simulink model "Ports"  (Simulink 7.4)
settings: Solver=ode45  StartTime=0.0  StopTime=10.0  RelTol=1e-3
settings Model: Creator=dread  LastModifiedBy=dread

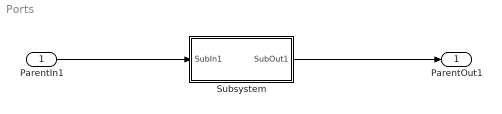
== system Ports ==
  ParentIn1 : Inport  OutDataType=fixdt(1, 16)  OutScaling=2^0
  Subsystem : Subsystem
  ParentOut1 : Outport  OutDataType=fixdt(1, 16)  OutScaling=2^0
  wires:
  ParentIn1/1 -> Subsystem/1(SubIn1)
  Subsystem/1(SubOut1) -> ParentOut1/1

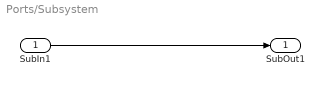
== system Ports/Subsystem ==
  SubIn1 : Inport  OutDataType=fixdt(1, 16)  OutScaling=2^0
  SubOut1 : Outport  OutDataType=fixdt(1, 16)  OutScaling=2^0
  wires:
  SubIn1/1 -> SubOut1/1
